simulink model "lqr_nlin"  (R2015a)
settings: Solver=ode45  StartTime=0.0  StopTime=30  FixedStep=6e-3  RelTol=1e-3
values from neighbouring files (symbols this model uses):
  A = [-inv(MP_bar)*CP_bar zeros(2,1) inv(MP_bar)*B_km;     -1/(Yl+Yr) 1/(Yl+Yr) zeros(1,3);     -Kbl*N/La 0 0 -Ra/La 0;     0 -Kbr*N/La 0 0 -Ra/La]    [Diseno_controlador_LQR_skid_steer.m]    (also in S_Rover_skid_steer.m = [-inv(M_b*P)*C_b*P zeros(2,1) inv(M_b*P)*B_b*Km;     -r/(Yl+)
  B = Kpwm/La*[zeros(3,2);eye(2)]    [Diseno_controlador_LQR_skid_steer.m]    (also in S_Rover_skid_steer.m = [zeros(3,2);Kpwm/La 0;0 Kpwm/La])
  Kc = Ka(:,1:5)    [Diseno_controlador_LQR_skid_steer.m]
  Ki = Ka(:,6:7)    [Diseno_controlador_LQR_skid_steer.m]
  Ts = 60e-3    (= 0.06)    [Diseno_controlador_LQR_skid_steer.m]
libraries: dspsrcs4 x2
settings Model: CovModelRefEnable=off  Creator=haroldfmurcia  LastModifiedBy=Juan_David
settings DataIOCC: SaveFormat=StructureWithTime
settings HardwareCC: ProdBitPerPointer=64  ProdLargestAtomicFloat=Float  ProdIntDivRoundTo=Zero  ProdEndianess=LittleEndian  ProdHWDeviceType=Specified
settings GRTTargetCC: GeneratePreprocessorConditionals=Use local settings

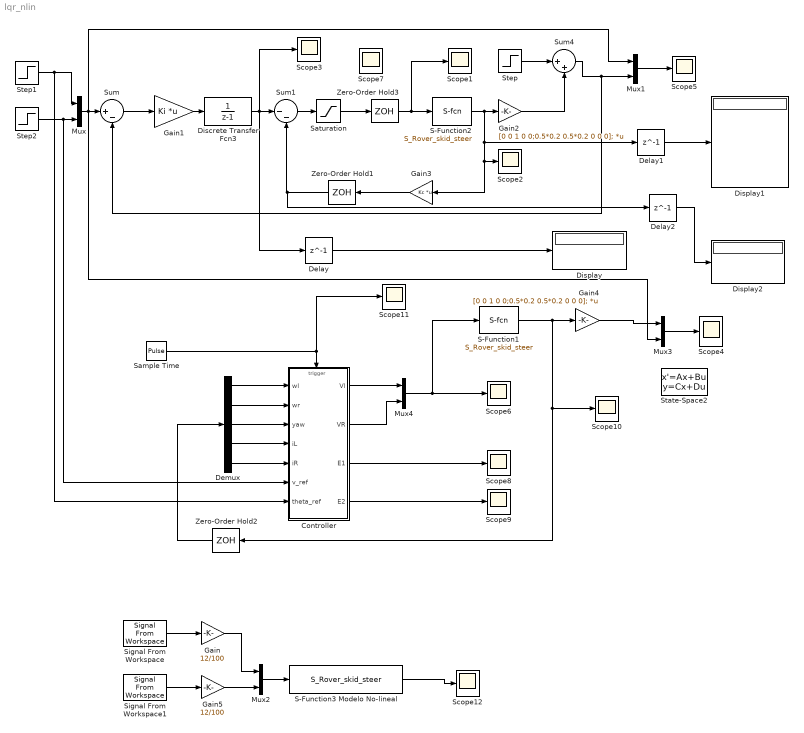
== system lqr_nlin ==
  Controller : Subsystem
  Delay : Delay  DelayLength=1  SampleTime=Ts
  Delay1 : Delay  DelayLength=1  SampleTime=Ts
  Delay2 : Delay  DelayLength=1  SampleTime=Ts
  Demux : Demux  Outputs=5
  Discrete Transfer Fcn3 : DiscreteTransferFcn  Denominator=[1 -1]  SampleTime=Ts
  Display : Display
  Display1 : Display
  Display2 : Display
  Gain : Gain  Gain=12/100
  Gain1 : Gain  Gain=Ki  Multiplication=Matrix(K*u) (u vector)
  Gain2 : Gain  Gain=[0 0 1 0 0;0.5*0.2 0.5*0.2 0 0 0];  Multiplication=Matrix(K*u) (u vector)  SampleTime=Ts
  Gain3 : Gain  Gain=Kc  Multiplication=Matrix(K*u) (u vector)
  Gain4 : Gain  Gain=[0 0 1 0 0;0.5*0.2 0.5*0.2 0 0 0];  Multiplication=Matrix(K*u) (u vector)  SampleTime=Ts
  Gain5 : Gain  Gain=12/100
  Mux{,1..4} (5 alike) : Mux  Inputs=2
  S-Function1 : S-Function  FunctionName=S_Rover_skid_steer
  S-Function2 : S-Function  FunctionName=S_Rover_skid_steer
  S-Function3 Modelo No-lineal : S-Function  FunctionName=S_Rover_skid_steer
  Sample Time : DiscretePulseGenerator  PulseType=Time based  Period=Ts  PulseWidth=10  SampleTime=1e-3
  Saturation : Saturate  UpperLimit=100  LowerLimit=-100
  Scope{1..12} (12 alike) : Scope
      Scope1 settings: YMin=-73.24295  YMax=119.24922
      Scope10 settings: YMin=-57.1366  YMax=46.62882  SaveName=ScopeData2
      Scope11 settings: YMin=-1.00000  YMax=1.00000  SaveName=ScopeData3
      Scope12 settings: YMin=-0.7  YMax=0.7  SaveName=ScopeData7
      Scope2 settings: YMin=-32.95456  YMax=24.9659
      Scope3 settings: YMin=-50.1371  YMax=63.52669  SaveName=ScopeData2
      Scope4 settings: YMin=-0.75  YMax=2.25  SaveName=ScopeData3  MaxDataPoints=500000
      Scope5 settings: YMin=-0.25  YMax=2.25  SaveName=ScopeData5  MaxDataPoints=500000
      Scope6 settings: YMin=-70  YMax=50  SaveName=ScopeData4  MaxDataPoints=500000
      Scope7 settings: YMin=-874.60938  YMax=857.62638  SaveName=ScopeData5
      Scope8 settings: YMin=-461.30149  YMax=379.73798  SaveName=ScopeData6
      Scope9 settings: YMin=-2.0067  YMax=5.27898
  Signal From Workspace : dspsrcs4/Signal From Workspace  X=U_Iz  Ts=Ts  nsamps=1  OutputAfterFinalValue=Setting to zero  ignoreOrWarnInputAndFrameLengths=off
  Signal From Workspace1 : dspsrcs4/Signal From Workspace  X=U_Der  Ts=Ts  nsamps=1  OutputAfterFinalValue=Setting to zero  ignoreOrWarnInputAndFrameLengths=off
  State-Space2 : StateSpace  A=A  B=B  C=eye(5)  D=zeros(5,2)  X0=0  ContinuousStateAttributes='position'
  Step : Step  Time=3  After=0  SampleTime=0
  Step1 : Step  Time=6  After=pi/2  SampleTime=0
  Step2 : Step  Time=5  Before=1  After=0  SampleTime=0
  Sum : Sum  Inputs=|+-
  Sum1 : Sum  Inputs=|--
  Sum4 : Sum  Inputs=|++
  Zero-Order Hold1 : ZeroOrderHold  SampleTime=Ts
  Zero-Order Hold2 : ZeroOrderHold  SampleTime=Ts
  Zero-Order Hold3 : ZeroOrderHold  SampleTime=Ts
  wires:
  Gain3/1 -> Zero-Order Hold1/1
  Gain2/1 -> Sum4/2
  Sum1/1 -> Saturation/1
  Sum4/1 -> Sum/2, Mux1/2
  Gain1/1 -> Discrete Transfer Fcn3/1
  Step1/1 -> Controller/7(theta_ref), Mux/1
  Step2/1 -> Controller/6(v_ref), Mux/2
  Mux1/1 -> Scope5/1
  S-Function2/1 -> Gain2/1, Delay1/1, Gain3/1, Scope2/1
  Step/1 -> Sum4/1
  Mux/1 -> Mux3/2, Mux1/1, Sum/1
  Mux3/1 -> Scope4/1
  Gain4/1 -> Mux3/1
  Sample Time/1 -> Controller/Trigger, Scope11/1
  Controller/1(Vl) -> Mux4/1
  Controller/2(VR) -> Mux4/2
  Demux/1 -> Controller/1(wl)
  Demux/2 -> Controller/2(wr)
  Demux/3 -> Controller/3(yaw)
  Demux/4 -> Controller/4(iL)
  Demux/5 -> Controller/5(iR)
  S-Function1/1 -> Gain4/1, Scope10/1, Zero-Order Hold2/1
  Controller/3(E1) -> Scope8/1
  Controller/4(E2) -> Scope9/1
  Mux4/1 -> S-Function1/1, Scope6/1
  Zero-Order Hold3/1 -> S-Function2/1, Scope1/1
  Sum/1 -> Gain1/1
  Zero-Order Hold2/1 -> Demux/1
  Zero-Order Hold1/1 -> Delay2/1, Sum1/2
  Discrete Transfer Fcn3/1 -> Scope3/1, Delay/1, Sum1/1
  Delay/1 -> Display/1
  Delay1/1 -> Display1/1
  Saturation/1 -> Zero-Order Hold3/1
  Delay2/1 -> Display2/1
  S-Function3 Modelo No-lineal/1 -> Scope12/1
  Mux2/1 -> S-Function3 Modelo No-lineal/1
  Signal From Workspace/1 -> Gain/1
  Signal From Workspace1/1 -> Gain5/1
  Gain5/1 -> Mux2/2
  Gain/1 -> Mux2/1

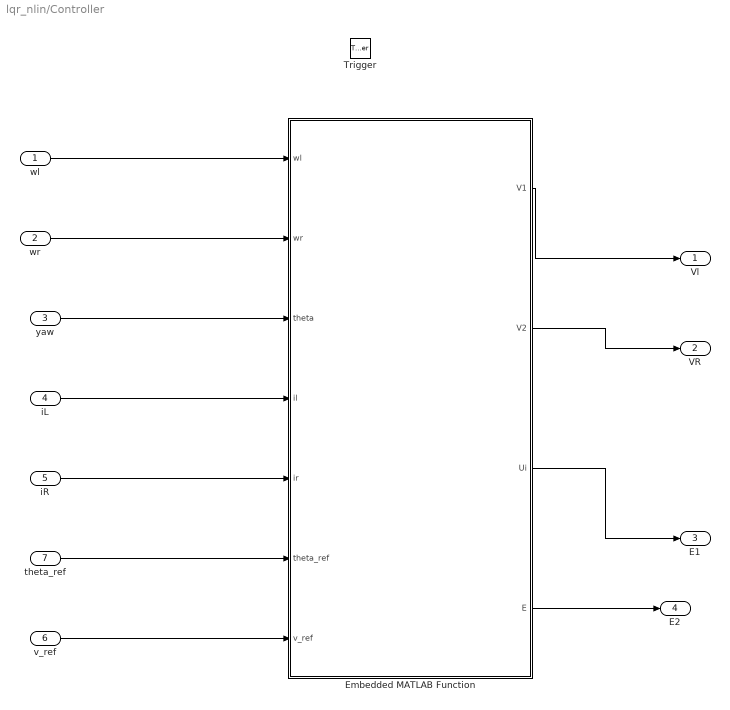
== system lqr_nlin/Controller ==
  wl : Inport
  wr : Inport  Port=2
  yaw : Inport  Port=3
  iL : Inport  Port=4
  iR : Inport  Port=5
  v_ref : Inport  Port=6
  theta_ref : Inport  Port=7
  Trigger : TriggerPort
  Embedded MATLAB Function : MATLAB Function  TreatAsAtomicUnit=on
  Vl : Outport
  VR : Outport  Port=2
  E1 : Outport  Port=3
  E2 : Outport  Port=4
  wires:
  Embedded MATLAB Function/1(V1) -> Vl/1
  wl/1 -> Embedded MATLAB Function/1(wl)
  wr/1 -> Embedded MATLAB Function/2(wr)
  Embedded MATLAB Function/2(V2) -> VR/1
  yaw/1 -> Embedded MATLAB Function/3(theta)
  theta_ref/1 -> Embedded MATLAB Function/6(theta_ref)
  v_ref/1 -> Embedded MATLAB Function/7(v_ref)
  Embedded MATLAB Function/3(Ui) -> E1/1
  Embedded MATLAB Function/4(E) -> E2/1
  iL/1 -> Embedded MATLAB Function/4(il)
  iR/1 -> Embedded MATLAB Function/5(ir)

== matlab function lqr_nlin/Controller/Embedded MATLAB Function ==
  data: wl input; V1 output; wr input; V2 output; theta input; il input; ir input; theta_ref input; v_ref input; Ui output; E output
function [V1,V2,Ui,E]  = fcn(wl,wr,theta,il,ir,theta_ref,v_ref)

 persistent Ui_1 E_1 Cd Ka;
% 
 if isempty(Ui_1);
     Ui_1=[0;0];   
 end;
 
 if isempty(E_1); 
     E_1=[0;0];   
 end;
 
 
  if isempty(Cd);
     Cd=zeros(2,5);   
 end;
 
  
  if isempty(Ka);
     Ka=zeros(2,7);   
 end;
 
 Ki=[5.4795   -6.1992;
   -4.9999   -4.8503];

%     13.0129212743297860 -3.173079275057106;
%    -12.186102519656009 -2.422711541551643];

Kc=[68.1353  -43.3090 -120.8227    3.3142   -0.5213;
  -38.5155   56.0487  106.4006   -0.3622    2.8937];
   % 0.902690451558094   -0.748439773175955  -2.162983641273786  0.034786670401752   -0.010597252888893;
   %-0.693575114318918   0.796801507499685   1.998622154232831   -0.007372139162157  0.031635979340854];

%% Parametros
Ts=60e-3;
w_l=wl;
w_r=wr;

I_l=il;
I_r=ir;

N=16;
r=0.2;
L=0.61/2;  %ancho del carro
a=0.62/2;  %Largo del carro
m=58;
Kpwm=0.1237;
g=9.81;
Yr=0.45;
Yl=Yr;
Kbr=0.0592;
Kbl=0.0637;
Kmr=0.0946;
Kml=0.0770;
Xg=-0.079; 
La= 0.081;
Ra=0.33;
I=15;
u_r=0.001;
u_l=0.8;
   

P=r/(Yl+Yr)*[Yr Yl;-1 1];
q_dot=P*[w_l;w_r];
x_dot=q_dot(1);
w_rover=q_dot(2);
y_dot=w_rover*Xg;

x1r_dot=x_dot-L*w_rover;
x2r_dot=x_dot+L*w_rover;
y1r_dot=y_dot+a*w_rover;
y3r_dot=y_dot-a*w_rover;
Rx=u_r*m*g/2*(sign(x1r_dot)+sign(x2r_dot));
Fy=u_l*m*g/2*(sign(y1r_dot)+sign(y3r_dot));
Mr=u_l*a*m*g/2*(sign(y1r_dot)-sign(y3r_dot))+u_r*L*m*g/2*(sign(x2r_dot)-sign(x1r_dot));


M_b=[m 0;...
     0 m*Xg^2+I];

C_b=m*Xg*w_rover*[0 1;-1 0];
R_b=[Rx*cos(theta)-Fy*sin(theta);...
     Xg*(Rx*sin(theta)+Fy*cos(theta))+Mr];
 
B_b=1/r*[1 1;-L L];

Km=N*[Kml 0;0 Kmr];

%% Dynamic matrix %%%%%%%%%%%%%%%%%%%%%%%%%%%%%%

A=[-inv(M_b*P)*C_b*P zeros(2,1) inv(M_b*P)*B_b*Km;...
    -r/(Yl+Yr) r/(Yl+Yr) zeros(1,3);...
    -Kbl*N/La 0 0 -Ra/La 0;...
    0 -Kbr*N/La 0 0 -Ra/La];

B=[zeros(3,2);Kpwm/La 0;0 Kpwm/La];

F=[inv(M_b*P)*R_b;zeros(3,1)];

C=[0 0 1 0 0;0.5*0.2 0.5*0.2 0 0 0];

D=zeros(2)

eml.extrinsic('ss');
eml.extrinsic('c2d');
eml.extrinsic('ssdata');
eml.extrinsic('dlqr');
ssc_rover=ss(A,B,C,D);

ssd_rover=c2d(ssc_rover,Ts);

[Ad,Bd,Cd,Dd,TS] = ssdata(ssd_rover) ;

 Ada=[Ad zeros(5,2);-Cd eye(2)];
 Bda=[Bd;zeros(2)];
 Cda=[Cd zeros(2)];
 Dda=zeros(2,2);
% 
 Q=diag([1 1 .1 1 1 2.25 1]);

 R=diag([0.04 0.06]);

 
Ka=dlqr(Ada,Bda,Q,R);
Kc=Ka(:,1:5);
Ki=Ka(:,6:7)

   %% CONTROL
    x=[wl;wr;theta;il;ir];
    C=[0 0 1 0 0;...
       0.5*0.2 0.5*0.2 0 0 0];
    Ref=[theta_ref;v_ref];
    E=Ref-C*x;
    Ui = (Ki*E_1)+Ui_1;
    Ut = -Ui-Kc*x;
    
    Ui_1=Ui;
    E_1=E;

if(Ut(1))>100
    Ut(1)=100;
elseif Ut(1)<-100
    Ut(1)=-100;
end

if(Ut(2))>100
    Ut(2)=100;
elseif Ut(2)<-100
    Ut(2)=-100;
end

V1=Ut(1);%;*100/12.1;
V2=Ut(2);%;*100/12.1;
